simulink model "templatePQreplay"  (R2019b)
settings: Solver=ode23tb  StartTime=0  StopTime=dataSim(l).Time(end)  FixedStep=Ts
model workspace (MAT data in the model file):
  AC8B_test_sdosession : sldodialogs.data.SessionData (value not decoded)
  tp34291882_bceb_4da8_b486_81ba615ab517 = [0 0.0333333 0.0666667 0.1 0.1333334 0.1666667 0.2 0.2333333 0.2666666 0.2999999 0.3333332 0.3666665 ... (13500 elements, 2700x5)]
  tp5fd81924_c6b2_4820_a4c1_c746ac51258e.time = 0
  tp5fd81924_c6b2_4820_a4c1_c746ac51258e.signals(1).values = 0.585108892137
  tp5fd81924_c6b2_4820_a4c1_c746ac51258e.signals(1).dimensions = 1
  tp5fd81924_c6b2_4820_a4c1_c746ac51258e.signals(1).label = 'CSTATE'
  tp5fd81924_c6b2_4820_a4c1_c746ac51258e.signals(1).blockName = 'Unit_I_GAS_AVR_PSS_GOV/General Governor
    | (Continuous)/Break
    | Algebraic
    | Loop /Integrator'
  tp5fd81924_c6b2_4820_a4c1_c746ac51258e.signals(1).stateName = ''
  tp5fd81924_c6b2_4820_a4c1_c746ac51258e.signals(1).inReferencedModel = 0
  tp5fd81924_c6b2_4820_a4c1_c746ac51258e.signals(1).sampleTime = [0 0]
  tp5fd81924_c6b2_4820_a4c1_c746ac51258e.signals(2).values = 0.50266340869
  tp5fd81924_c6b2_4820_a4c1_c746ac51258e.signals(2).dimensions = 1
  tp5fd81924_c6b2_4820_a4c1_c746ac51258e.signals(2).label = 'CSTATE'
  tp5fd81924_c6b2_4820_a4c1_c746ac51258e.signals(2).blockName = 'Unit_I_GAS_AVR_PSS_GOV/General Governor
    | (Continuous)/S0/Integrator'
  tp5fd81924_c6b2_4820_a4c1_c746ac51258e.signals(2).stateName = ''
  tp5fd81924_c6b2_4820_a4c1_c746ac51258e.signals(2).inReferencedModel = 0
  tp5fd81924_c6b2_4820_a4c1_c746ac51258e.signals(2).sampleTime = [0 0]
  tp5fd81924_c6b2_4820_a4c1_c746ac51258e.signals(3).values = -4.9502276038e-07
  tp5fd81924_c6b2_4820_a4c1_c746ac51258e.signals(3).dimensions = 1
  tp5fd81924_c6b2_4820_a4c1_c746ac51258e.signals(3).label = 'CSTATE'
  tp5fd81924_c6b2_4820_a4c1_c746ac51258e.signals(3).blockName = 'Unit_I_GAS_AVR_PSS_GOV/General Governor
    | (Continuous)/S1/S1_TF/Integrator'
  tp5fd81924_c6b2_4820_a4c1_c746ac51258e.signals(3).stateName = ''
  tp5fd81924_c6b2_4820_a4c1_c746ac51258e.signals(3).inReferencedModel = 0
  tp5fd81924_c6b2_4820_a4c1_c746ac51258e.signals(3).sampleTime = [0 0]
  tp5fd81924_c6b2_4820_a4c1_c746ac51258e.signals(4).values = 0.585110202145
  tp5fd81924_c6b2_4820_a4c1_c746ac51258e.signals(4).dimensions = 1
  tp5fd81924_c6b2_4820_a4c1_c746ac51258e.signals(4).label = 'CSTATE'
  tp5fd81924_c6b2_4820_a4c1_c746ac51258e.signals(4).blockName = 'Unit_I_GAS_AVR_PSS_GOV/General Governor
    | (Continuous)/S2/Integrator'
  tp5fd81924_c6b2_4820_a4c1_c746ac51258e.signals(4).stateName = ''
  tp5fd81924_c6b2_4820_a4c1_c746ac51258e.signals(4).inReferencedModel = 0
  tp5fd81924_c6b2_4820_a4c1_c746ac51258e.signals(4).sampleTime = [0 0]
  tp5fd81924_c6b2_4820_a4c1_c746ac51258e.signals(5).values = 0.585108893326
  tp5fd81924_c6b2_4820_a4c1_c746ac51258e.signals(5).dimensions = 1
  tp5fd81924_c6b2_4820_a4c1_c746ac51258e.signals(5).label = 'CSTATE'
  tp5fd81924_c6b2_4820_a4c1_c746ac51258e.signals(5).blockName = 'Unit_I_GAS_AVR_PSS_GOV/General Governor
    | (Continuous)/S3/Integrator'
  tp5fd81924_c6b2_4820_a4c1_c746ac51258e.signals(5).stateName = ''
  tp5fd81924_c6b2_4820_a4c1_c746ac51258e.signals(5).inReferencedModel = 0
  tp5fd81924_c6b2_4820_a4c1_c746ac51258e.signals(5).sampleTime = [0 0]
  tp5fd81924_c6b2_4820_a4c1_c746ac51258e.signals(6).values = 0.502663324956
  tp5fd81924_c6b2_4820_a4c1_c746ac51258e.signals(6).dimensions = 1
  tp5fd81924_c6b2_4820_a4c1_c746ac51258e.signals(6).label = 'CSTATE'
  tp5fd81924_c6b2_4820_a4c1_c746ac51258e.signals(6).blockName = 'Unit_I_GAS_AVR_PSS_GOV/General Governor
    | (Continuous)/S4/Integrator'
  tp5fd81924_c6b2_4820_a4c1_c746ac51258e.signals(6).stateName = ''
  tp5fd81924_c6b2_4820_a4c1_c746ac51258e.signals(6).inReferencedModel = 0
  tp5fd81924_c6b2_4820_a4c1_c746ac51258e.signals(6).sampleTime = [0 0]
  tp5fd81924_c6b2_4820_a4c1_c746ac51258e.signals(7).values = 0.585108883007
  tp5fd81924_c6b2_4820_a4c1_c746ac51258e.signals(7).dimensions = 1
  tp5fd81924_c6b2_4820_a4c1_c746ac51258e.signals(7).label = 'CSTATE'
  tp5fd81924_c6b2_4820_a4c1_c746ac51258e.signals(7).blockName = 'Unit_I_GAS_AVR_PSS_GOV/General Governor
    | (Continuous)/S5/Integrator'
  tp5fd81924_c6b2_4820_a4c1_c746ac51258e.signals(7).stateName = ''
  tp5fd81924_c6b2_4820_a4c1_c746ac51258e.signals(7).inReferencedModel = 0
  tp5fd81924_c6b2_4820_a4c1_c746ac51258e.signals(7).sampleTime = [0 0]
  tp5fd81924_c6b2_4820_a4c1_c746ac51258e.signals(8).values = 0.585108892137
  tp5fd81924_c6b2_4820_a4c1_c746ac51258e.signals(8).dimensions = 1
  tp5fd81924_c6b2_4820_a4c1_c746ac51258e.signals(8).label = 'CSTATE'
  tp5fd81924_c6b2_4820_a4c1_c746ac51258e.signals(8).blockName = 'Unit_I_GAS_AVR_PSS_GOV/General Governor
    | (Continuous)/S6/Integrator'
  tp5fd81924_c6b2_4820_a4c1_c746ac51258e.signals(8).stateName = ''
  tp5fd81924_c6b2_4820_a4c1_c746ac51258e.signals(8).inReferencedModel = 0
  tp5fd81924_c6b2_4820_a4c1_c746ac51258e.signals(8).sampleTime = [0 0]
  tp5fd81924_c6b2_4820_a4c1_c746ac51258e.signals(9).values = 0.0335271378154
  tp5fd81924_c6b2_4820_a4c1_c746ac51258e.signals(9).dimensions = 1
  tp5fd81924_c6b2_4820_a4c1_c746ac51258e.signals(9).label = 'CSTATE'
  tp5fd81924_c6b2_4820_a4c1_c746ac51258e.signals(9).blockName = 'Unit_I_GAS_AVR_PSS_GOV/General Governor
    | (Continuous)/S7/Integrator'
  tp5fd81924_c6b2_4820_a4c1_c746ac51258e.signals(9).stateName = ''
  tp5fd81924_c6b2_4820_a4c1_c746ac51258e.signals(9).inReferencedModel = 0
  tp5fd81924_c6b2_4820_a4c1_c746ac51258e.signals(9).sampleTime = [0 0]
  tp5fd81924_c6b2_4820_a4c1_c746ac51258e.signals(10).values = -1.76344898171e-08
  tp5fd81924_c6b2_4820_a4c1_c746ac51258e.signals(10).dimensions = 1
  tp5fd81924_c6b2_4820_a4c1_c746ac51258e.signals(10).label = 'CSTATE'
  tp5fd81924_c6b2_4820_a4c1_c746ac51258e.signals(10).blockName = 'Unit_I_GAS_AVR_PSS_GOV/General Governor
    | (Continuous)/S8/Integrator'
  tp5fd81924_c6b2_4820_a4c1_c746ac51258e.signals(10).stateName = ''
  tp5fd81924_c6b2_4820_a4c1_c746ac51258e.signals(10).inReferencedModel = 0
  tp5fd81924_c6b2_4820_a4c1_c746ac51258e.signals(10).sampleTime = [0 0]
  tp5fd81924_c6b2_4820_a4c1_c746ac51258e.signals(11).values = 0.585108883007
  tp5fd81924_c6b2_4820_a4c1_c746ac51258e.signals(11).dimensions = 1
  tp5fd81924_c6b2_4820_a4c1_c746ac51258e.signals(11).label = 'CSTATE'
  tp5fd81924_c6b2_4820_a4c1_c746ac51258e.signals(11).blockName = 'Unit_I_GAS_AVR_PSS_GOV/General Governor
    | (Continuous)/S9/Integrator'
  tp5fd81924_c6b2_4820_a4c1_c746ac51258e.signals(11).stateName = ''
  tp5fd81924_c6b2_4820_a4c1_c746ac51258e.signals(11).inReferencedModel = 0
  tp5fd81924_c6b2_4820_a4c1_c746ac51258e.signals(11).sampleTime = [0 0]
  tp5fd81924_c6b2_4820_a4c1_c746ac51258e.signals(12).values = 1.09585681999
  tp5fd81924_c6b2_4820_a4c1_c746ac51258e.signals(12).dimensions = 1
  tp5fd81924_c6b2_4820_a4c1_c746ac51258e.signals(12).label = 'CSTATE'
  tp5fd81924_c6b2_4820_a4c1_c746ac51258e.signals(12).blockName = 'Unit_I_GAS_AVR_PSS_GOV/General Purpose
    | Rotating Excitation System
    | (Continuous)/S0/Tr ~= 0/Integrator'
  tp5fd81924_c6b2_4820_a4c1_c746ac51258e.signals(12).stateName = ''
  tp5fd81924_c6b2_4820_a4c1_c746ac51258e.signals(12).inReferencedModel = 0
  tp5fd81924_c6b2_4820_a4c1_c746ac51258e.signals(12).sampleTime = [0 0]
  tp5fd81924_c6b2_4820_a4c1_c746ac51258e.signals(13).values = -1.11082263543e-06
  tp5fd81924_c6b2_4820_a4c1_c746ac51258e.signals(13).dimensions = 1
  tp5fd81924_c6b2_4820_a4c1_c746ac51258e.signals(13).label = 'CSTATE'
  tp5fd81924_c6b2_4820_a4c1_c746ac51258e.signals(13).blockName = 'Unit_I_GAS_AVR_PSS_GOV/General Purpose
    | Rotating Excitation System
    | (Continuous)/S1/Integrator'
  tp5fd81924_c6b2_4820_a4c1_c746ac51258e.signals(13).stateName = ''
  tp5fd81924_c6b2_4820_a4c1_c746ac51258e.signals(13).inReferencedModel = 0
  tp5fd81924_c6b2_4820_a4c1_c746ac51258e.signals(13).sampleTime = [0 0]
  tp5fd81924_c6b2_4820_a4c1_c746ac51258e.signals(14).values = 0.294440520333
  tp5fd81924_c6b2_4820_a4c1_c746ac51258e.signals(14).dimensions = 1
  tp5fd81924_c6b2_4820_a4c1_c746ac51258e.signals(14).label = 'CSTATE'
  tp5fd81924_c6b2_4820_a4c1_c746ac51258e.signals(14).blockName = 'Unit_I_GAS_AVR_PSS_GOV/General Purpose
    | Rotating Excitation System
    | (Continuous)/S2 + S8/S2/Tb1 ~= 0/Integrator'
  tp5fd81924_c6b2_4820_a4c1_c746ac51258e.signals(14).stateName = ''
  tp5fd81924_c6b2_4820_a4c1_c746ac51258e.signals(14).inReferencedModel = 0
  tp5fd81924_c6b2_4820_a4c1_c746ac51258e.signals(14).sampleTime = [0 0]
  tp5fd81924_c6b2_4820_a4c1_c746ac51258e.signals(15).values = 0.294440505746
  tp5fd81924_c6b2_4820_a4c1_c746ac51258e.signals(15).dimensions = 1
  tp5fd81924_c6b2_4820_a4c1_c746ac51258e.signals(15).label = 'CSTATE'
  tp5fd81924_c6b2_4820_a4c1_c746ac51258e.signals(15).blockName = 'Unit_I_GAS_AVR_PSS_GOV/General Purpose
    | Rotating Excitation System
    | (Continuous)/S2 + S8/S8/Tb2 ~= 0/Integrator'
  tp5fd81924_c6b2_4820_a4c1_c746ac51258e.signals(15).stateName = ''
  tp5fd81924_c6b2_4820_a4c1_c746ac51258e.signals(15).inReferencedModel = 0
  tp5fd81924_c6b2_4820_a4c1_c746ac51258e.signals(15).sampleTime = [0 0]
  tp5fd81924_c6b2_4820_a4c1_c746ac51258e.signals(16).values = 0.29444050528
  tp5fd81924_c6b2_4820_a4c1_c746ac51258e.signals(16).dimensions = 1
  tp5fd81924_c6b2_4820_a4c1_c746ac51258e.signals(16).label = 'CSTATE'
  tp5fd81924_c6b2_4820_a4c1_c746ac51258e.signals(16).blockName = 'Unit_I_GAS_AVR_PSS_GOV/General Purpose
    | Rotating Excitation System
    | (Continuous)/S3/Ta ~= 0/Integrator'
  tp5fd81924_c6b2_4820_a4c1_c746ac51258e.signals(16).stateName = ''
  tp5fd81924_c6b2_4820_a4c1_c746ac51258e.signals(16).inReferencedModel = 0
  tp5fd81924_c6b2_4820_a4c1_c746ac51258e.signals(16).sampleTime = [0 0]
  tp5fd81924_c6b2_4820_a4c1_c746ac51258e.signals(17).values = 1.17292432998
  tp5fd81924_c6b2_4820_a4c1_c746ac51258e.signals(17).dimensions = 1
  tp5fd81924_c6b2_4820_a4c1_c746ac51258e.signals(17).label = 'CSTATE'
  tp5fd81924_c6b2_4820_a4c1_c746ac51258e.signals(17).blockName = 'Unit_I_GAS_AVR_PSS_GOV/General Purpose
    | Rotating Excitation System
    | (Continuous)/S4/Tf2 ~= 0/Integrator'
  tp5fd81924_c6b2_4820_a4c1_c746ac51258e.signals(17).stateName = ''
  tp5fd81924_c6b2_4820_a4c1_c746ac51258e.signals(17).inReferencedModel = 0
  tp5fd81924_c6b2_4820_a4c1_c746ac51258e.signals(17).sampleTime = [0 0]
  tp5fd81924_c6b2_4820_a4c1_c746ac51258e.signals(18).values = 1.17292433904
  tp5fd81924_c6b2_4820_a4c1_c746ac51258e.signals(18).dimensions = 1
  tp5fd81924_c6b2_4820_a4c1_c746ac51258e.signals(18).label = 'CSTATE'
  tp5fd81924_c6b2_4820_a4c1_c746ac51258e.signals(18).blockName = 'Unit_I_GAS_AVR_PSS_GOV/General Purpose
    | Rotating Excitation System
    | (Continuous)/S5/Integrator'
  tp5fd81924_c6b2_4820_a4c1_c746ac51258e.signals(18).stateName = ''
  tp5fd81924_c6b2_4820_a4c1_c746ac51258e.signals(18).inReferencedModel = 0
  tp5fd81924_c6b2_4820_a4c1_c746ac51258e.signals(18).sampleTime = [0 0]
  tp5fd81924_c6b2_4820_a4c1_c746ac51258e.signals(19).values = -0.299278194471
  tp5fd81924_c6b2_4820_a4c1_c746ac51258e.signals(19).dimensions = 1
  tp5fd81924_c6b2_4820_a4c1_c746ac51258e.signals(19).label = 'CSTATE'
  tp5fd81924_c6b2_4820_a4c1_c746ac51258e.signals(19).blockName = 'Unit_I_GAS_AVR_PSS_GOV/General Purpose
    | Rotating Excitation System
    | (Continuous)/S6/Integrator'
  tp5fd81924_c6b2_4820_a4c1_c746ac51258e.signals(19).stateName = ''
  tp5fd81924_c6b2_4820_a4c1_c746ac51258e.signals(19).inReferencedModel = 0
  tp5fd81924_c6b2_4820_a4c1_c746ac51258e.signals(19).sampleTime = [0 0]
  tp5fd81924_c6b2_4820_a4c1_c746ac51258e.signals(20).values = 1.50129144782
  tp5fd81924_c6b2_4820_a4c1_c746ac51258e.signals(20).dimensions = 1
  tp5fd81924_c6b2_4820_a4c1_c746ac51258e.signals(20).label = 'CSTATE'
  tp5fd81924_c6b2_4820_a4c1_c746ac51258e.signals(20).blockName = 'Unit_I_GAS_AVR_PSS_GOV/General Purpose
    | Rotating Excitation System
    | (Continuous)/S7/Integrator'
  tp5fd81924_c6b2_4820_a4c1_c746ac51258e.signals(20).stateName = ''
  tp5fd81924_c6b2_4820_a4c1_c746ac51258e.signals(20).inReferencedModel = 0
  tp5fd81924_c6b2_4820_a4c1_c746ac51258e.signals(20).sampleTime = [0 0]
  tp5fd81924_c6b2_4820_a4c1_c746ac51258e.signals(21).values = 1.17292433193
  tp5fd81924_c6b2_4820_a4c1_c746ac51258e.signals(21).dimensions = 1
  tp5fd81924_c6b2_4820_a4c1_c746ac51258e.signals(21).label = 'CSTATE'
  tp5fd81924_c6b2_4820_a4c1_c746ac51258e.signals(21).blockName = 'Unit_I_GAS_AVR_PSS_GOV/General Purpose
    | Rotating Excitation System
    | (Continuous)/S9/Tp ~= 0/Integrator'
  tp5fd81924_c6b2_4820_a4c1_c746ac51258e.signals(21).stateName = ''
  tp5fd81924_c6b2_4820_a4c1_c746ac51258e.signals(21).inReferencedModel = 0
  tp5fd81924_c6b2_4820_a4c1_c746ac51258e.signals(21).sampleTime = [0 0]
  tp5fd81924_c6b2_4820_a4c1_c746ac51258e.signals(22).values = -1.49881455181e-10
  tp5fd81924_c6b2_4820_a4c1_c746ac51258e.signals(22).dimensions = 1
  tp5fd81924_c6b2_4820_a4c1_c746ac51258e.signals(22).label = 'CSTATE'
  tp5fd81924_c6b2_4820_a4c1_c746ac51258e.signals(22).blockName = 'Unit_I_GAS_AVR_PSS_GOV/Power System
    | Stabilizer 2A
    | (Continuous)/Ramp-Tracking Filter/T9 ~= 0/Filter1/TF1/Integrator'
  tp5fd81924_c6b2_4820_a4c1_c746ac51258e.signals(22).stateName = ''
  tp5fd81924_c6b2_4820_a4c1_c746ac51258e.signals(22).inReferencedModel = 0
  tp5fd81924_c6b2_4820_a4c1_c746ac51258e.signals(22).sampleTime = [0 0]
  tp5fd81924_c6b2_4820_a4c1_c746ac51258e.signals(23).values = -1.50085906522e-10
  tp5fd81924_c6b2_4820_a4c1_c746ac51258e.signals(23).dimensions = 1
  tp5fd81924_c6b2_4820_a4c1_c746ac51258e.signals(23).label = 'CSTATE'
  tp5fd81924_c6b2_4820_a4c1_c746ac51258e.signals(23).blockName = 'Unit_I_GAS_AVR_PSS_GOV/Power System
    | Stabilizer 2A
    | (Continuous)/Ramp-Tracking Filter/T9 ~= 0/Filter1/TF2/Integrator'
  tp5fd81924_c6b2_4820_a4c1_c746ac51258e.signals(23).stateName = ''
  tp5fd81924_c6b2_4820_a4c1_c746ac51258e.signals(23).inReferencedModel = 0
  tp5fd81924_c6b2_4820_a4c1_c746ac51258e.signals(23).sampleTime = [0 0]
  tp5fd81924_c6b2_4820_a4c1_c746ac51258e.signals(24).values = -1.50034793802e-10
  tp5fd81924_c6b2_4820_a4c1_c746ac51258e.signals(24).dimensions = 1
  tp5fd81924_c6b2_4820_a4c1_c746ac51258e.signals(24).label = 'CSTATE'
  tp5fd81924_c6b2_4820_a4c1_c746ac51258e.signals(24).blockName = 'Unit_I_GAS_AVR_PSS_GOV/Power System
    | Stabilizer 2A
    | (Continuous)/Ramp-Tracking Filter/T9 ~= 0/Filter1/TF3/Integrator'
  tp5fd81924_c6b2_4820_a4c1_c746ac51258e.signals(24).stateName = ''
  tp5fd81924_c6b2_4820_a4c1_c746ac51258e.signals(24).inReferencedModel = 0
  tp5fd81924_c6b2_4820_a4c1_c746ac51258e.signals(24).sampleTime = [0 0]
  tp5fd81924_c6b2_4820_a4c1_c746ac51258e.signals(25).values = -1.49983681133e-10
  tp5fd81924_c6b2_4820_a4c1_c746ac51258e.signals(25).dimensions = 1
  tp5fd81924_c6b2_4820_a4c1_c746ac51258e.signals(25).label = 'CSTATE'
  tp5fd81924_c6b2_4820_a4c1_c746ac51258e.signals(25).blockName = 'Unit_I_GAS_AVR_PSS_GOV/Power System
    | Stabilizer 2A
    | (Continuous)/Ramp-Tracking Filter/T9 ~= 0/Filter1/TF4/Integrator'
  tp5fd81924_c6b2_4820_a4c1_c746ac51258e.signals(25).stateName = ''
  tp5fd81924_c6b2_4820_a4c1_c746ac51258e.signals(25).inReferencedModel = 0
  tp5fd81924_c6b2_4820_a4c1_c746ac51258e.signals(25).sampleTime = [0 0]
  tp5fd81924_c6b2_4820_a4c1_c746ac51258e.signals(26).values = -1.49932568515e-10
  tp5fd81924_c6b2_4820_a4c1_c746ac51258e.signals(26).dimensions = 1
  tp5fd81924_c6b2_4820_a4c1_c746ac51258e.signals(26).label = 'CSTATE'
  tp5fd81924_c6b2_4820_a4c1_c746ac51258e.signals(26).blockName = 'Unit_I_GAS_AVR_PSS_GOV/Power System
    | Stabilizer 2A
    | (Continuous)/Ramp-Tracking Filter/T9 ~= 0/Filter1/TF5/Integrator'
  tp5fd81924_c6b2_4820_a4c1_c746ac51258e.signals(26).stateName = ''
  tp5fd81924_c6b2_4820_a4c1_c746ac51258e.signals(26).inReferencedModel = 0
  tp5fd81924_c6b2_4820_a4c1_c746ac51258e.signals(26).sampleTime = [0 0]
  tp5fd81924_c6b2_4820_a4c1_c746ac51258e.signals(27).values = -1.76344805856e-08
  tp5fd81924_c6b2_4820_a4c1_c746ac51258e.signals(27).dimensions = 1
  tp5fd81924_c6b2_4820_a4c1_c746ac51258e.signals(27).label = 'CSTATE'
  tp5fd81924_c6b2_4820_a4c1_c746ac51258e.signals(27).blockName = 'Unit_I_GAS_AVR_PSS_GOV/Power System
    | Stabilizer 2A
    | (Continuous)/S0/Integrator'
  tp5fd81924_c6b2_4820_a4c1_c746ac51258e.signals(27).stateName = ''
  tp5fd81924_c6b2_4820_a4c1_c746ac51258e.signals(27).inReferencedModel = 0
  tp5fd81924_c6b2_4820_a4c1_c746ac51258e.signals(27).sampleTime = [0 0]
  tp5fd81924_c6b2_4820_a4c1_c746ac51258e.signals(28).values = 1.49872449229e-10
  tp5fd81924_c6b2_4820_a4c1_c746ac51258e.signals(28).dimensions = 1
  tp5fd81924_c6b2_4820_a4c1_c746ac51258e.signals(28).label = 'CSTATE'
  tp5fd81924_c6b2_4820_a4c1_c746ac51258e.signals(28).blockName = 'Unit_I_GAS_AVR_PSS_GOV/Power System
    | Stabilizer 2A
    | (Continuous)/S1/Tw2 ~= 0/Integrator'
  tp5fd81924_c6b2_4820_a4c1_c746ac51258e.signals(28).stateName = ''
  tp5fd81924_c6b2_4820_a4c1_c746ac51258e.signals(28).inReferencedModel = 0
  tp5fd81924_c6b2_4820_a4c1_c746ac51258e.signals(28).sampleTime = [0 0]
  tp5fd81924_c6b2_4820_a4c1_c746ac51258e.signals(29).values = -4.09162771813e-09
  tp5fd81924_c6b2_4820_a4c1_c746ac51258e.signals(29).dimensions = 1
  tp5fd81924_c6b2_4820_a4c1_c746ac51258e.signals(29).label = 'CSTATE'
  tp5fd81924_c6b2_4820_a4c1_c746ac51258e.signals(29).blockName = 'Unit_I_GAS_AVR_PSS_GOV/Power System
    | Stabilizer 2A
    | (Continuous)/S18/Tb ~= 0/Integrator'
  tp5fd81924_c6b2_4820_a4c1_c746ac51258e.signals(29).stateName = ''
  tp5fd81924_c6b2_4820_a4c1_c746ac51258e.signals(29).inReferencedModel = 0
  tp5fd81924_c6b2_4820_a4c1_c746ac51258e.signals(29).sampleTime = [0 0]
  tp5fd81924_c6b2_4820_a4c1_c746ac51258e.signals(30).values = -1.49882113433e-10
  tp5fd81924_c6b2_4820_a4c1_c746ac51258e.signals(30).dimensions = 1
  tp5fd81924_c6b2_4820_a4c1_c746ac51258e.signals(30).label = 'CSTATE'
  tp5fd81924_c6b2_4820_a4c1_c746ac51258e.signals(30).blockName = 'Unit_I_GAS_AVR_PSS_GOV/Power System
    | Stabilizer 2A
    | (Continuous)/S2/T6 ~= 0/Integrator'
  tp5fd81924_c6b2_4820_a4c1_c746ac51258e.signals(30).stateName = ''
  tp5fd81924_c6b2_4820_a4c1_c746ac51258e.signals(30).inReferencedModel = 0
  tp5fd81924_c6b2_4820_a4c1_c746ac51258e.signals(30).sampleTime = [0 0]
  tp5fd81924_c6b2_4820_a4c1_c746ac51258e.signals(31).values = 0.502663409208
  tp5fd81924_c6b2_4820_a4c1_c746ac51258e.signals(31).dimensions = 1
  tp5fd81924_c6b2_4820_a4c1_c746ac51258e.signals(31).label = 'CSTATE'
  tp5fd81924_c6b2_4820_a4c1_c746ac51258e.signals(31).blockName = 'Unit_I_GAS_AVR_PSS_GOV/Power System
    | Stabilizer 2A
    | (Continuous)/S3/Integrator'
  tp5fd81924_c6b2_4820_a4c1_c746ac51258e.signals(31).stateName = ''
  tp5fd81924_c6b2_4820_a4c1_c746ac51258e.signals(31).inReferencedModel = 0
  tp5fd81924_c6b2_4820_a4c1_c746ac51258e.signals(31).sampleTime = [0 0]
  tp5fd81924_c6b2_4820_a4c1_c746ac51258e.signals(32).values = -6.11813281183e-12
  tp5fd81924_c6b2_4820_a4c1_c746ac51258e.signals(32).dimensions = 1
  tp5fd81924_c6b2_4820_a4c1_c746ac51258e.signals(32).label = 'CSTATE'
  tp5fd81924_c6b2_4820_a4c1_c746ac51258e.signals(32).blockName = 'Unit_I_GAS_AVR_PSS_GOV/Power System
    | Stabilizer 2A
    | (Continuous)/S4/Tw4 ~= 0/Integrator'
  tp5fd81924_c6b2_4820_a4c1_c746ac51258e.signals(32).stateName = ''
  tp5fd81924_c6b2_4820_a4c1_c746ac51258e.signals(32).inReferencedModel = 0
  tp5fd81924_c6b2_4820_a4c1_c746ac51258e.signals(32).sampleTime = [0 0]
  tp5fd81924_c6b2_4820_a4c1_c746ac51258e.signals(33).values = 6.57485586185e-16
  tp5fd81924_c6b2_4820_a4c1_c746ac51258e.signals(33).dimensions = 1
  tp5fd81924_c6b2_4820_a4c1_c746ac51258e.signals(33).label = 'CSTATE'
  tp5fd81924_c6b2_4820_a4c1_c746ac51258e.signals(33).blockName = 'Unit_I_GAS_AVR_PSS_GOV/Power System
    | Stabilizer 2A
    | (Continuous)/S5/T7 ~= 0/Integrator'
  tp5fd81924_c6b2_4820_a4c1_c746ac51258e.signals(33).stateName = ''
  tp5fd81924_c6b2_4820_a4c1_c746ac51258e.signals(33).inReferencedModel = 0
  tp5fd81924_c6b2_4820_a4c1_c746ac51258e.signals(33).sampleTime = [0 0]
  tp5fd81924_c6b2_4820_a4c1_c746ac51258e.signals(34).values = -4.09146911874e-09
  tp5fd81924_c6b2_4820_a4c1_c746ac51258e.signals(34).dimensions = 1
  tp5fd81924_c6b2_4820_a4c1_c746ac51258e.signals(34).label = 'CSTATE'
  tp5fd81924_c6b2_4820_a4c1_c746ac51258e.signals(34).blockName = 'Unit_I_GAS_AVR_PSS_GOV/Power System
    | Stabilizer 2A
    | (Continuous)/S6/T2 ~= 0/Integrator'
  tp5fd81924_c6b2_4820_a4c1_c746ac51258e.signals(34).stateName = ''
  tp5fd81924_c6b2_4820_a4c1_c746ac51258e.signals(34).inReferencedModel = 0
  tp5fd81924_c6b2_4820_a4c1_c746ac51258e.signals(34).sampleTime = [0 0]
  tp5fd81924_c6b2_4820_a4c1_c746ac51258e.signals(35).values = -4.09167395604e-09
  tp5fd81924_c6b2_4820_a4c1_c746ac51258e.signals(35).dimensions = 1
  tp5fd81924_c6b2_4820_a4c1_c746ac51258e.signals(35).label = 'CSTATE'
  tp5fd81924_c6b2_4820_a4c1_c746ac51258e.signals(35).blockName = 'Unit_I_GAS_AVR_PSS_GOV/Power System
    | Stabilizer 2A
    | (Continuous)/S7/T4 ~= 0/Integrator'
  tp5fd81924_c6b2_4820_a4c1_c746ac51258e.signals(35).stateName = ''
  tp5fd81924_c6b2_4820_a4c1_c746ac51258e.signals(35).inReferencedModel = 0
  tp5fd81924_c6b2_4820_a4c1_c746ac51258e.signals(35).sampleTime = [0 0]
  tp5fd81924_c6b2_4820_a4c1_c746ac51258e.signals(36).values = 0.001094934692
  tp5fd81924_c6b2_4820_a4c1_c746ac51258e.signals(36).dimensions = 1
  tp5fd81924_c6b2_4820_a4c1_c746ac51258e.signals(36).label = 'CSTATE'
  tp5fd81924_c6b2_4820_a4c1_c746ac51258e.signals(36).blockName = 'Unit_I_GAS_AVR_PSS_GOV/Subsystem/Three-Phase
    | Dynamic Load/Model/ filter1'
  tp5fd81924_c6b2_4820_a4c1_c746ac51258e.signals(36).stateName = ''
  tp5fd81924_c6b2_4820_a4c1_c746ac51258e.signals(36).inReferencedModel = 0
  tp5fd81924_c6b2_4820_a4c1_c746ac51258e.signals(36).sampleTime = [0 0]
  tp5fd81924_c6b2_4820_a4c1_c746ac51258e.signals(37).values = 0.187748964781
  tp5fd81924_c6b2_4820_a4c1_c746ac51258e.signals(37).dimensions = 1
  tp5fd81924_c6b2_4820_a4c1_c746ac51258e.signals(37).label = 'CSTATE'
  tp5fd81924_c6b2_4820_a4c1_c746ac51258e.signals(37).blockName = 'Unit_I_GAS_AVR_PSS_GOV/Subsystem/Three-Phase
    | Dynamic Load/Model/Break 
    | Alg. Loop I1/imag/State Space'
  tp5fd81924_c6b2_4820_a4c1_c746ac51258e.signals(37).stateName = ''
  tp5fd81924_c6b2_4820_a4c1_c746ac51258e.signals(37).inReferencedModel = 0
  tp5fd81924_c6b2_4820_a4c1_c746ac51258e.signals(37).sampleTime = [0 0]
  tp5fd81924_c6b2_4820_a4c1_c746ac51258e.signals(38).values = -0.851179474107
  tp5fd81924_c6b2_4820_a4c1_c746ac51258e.signals(38).dimensions = 1
  tp5fd81924_c6b2_4820_a4c1_c746ac51258e.signals(38).label = 'CSTATE'
  tp5fd81924_c6b2_4820_a4c1_c746ac51258e.signals(38).blockName = 'Unit_I_GAS_AVR_PSS_GOV/Subsystem/Three-Phase
    | Dynamic Load/Model/Break 
    | Alg. Loop I1/real/State Space'
  tp5fd81924_c6b2_4820_a4c1_c746ac51258e.signals(38).stateName = ''
  tp5fd81924_c6b2_4820_a4c1_c746ac51258e.signals(38).inReferencedModel = 0
  tp5fd81924_c6b2_4820_a4c1_c746ac51258e.signals(38).sampleTime = [0 0]
  tp5fd81924_c6b2_4820_a4c1_c746ac51258e.signals(39).values = 0
  tp5fd81924_c6b2_4820_a4c1_c746ac51258e.signals(39).dimensions = 1
  tp5fd81924_c6b2_4820_a4c1_c746ac51258e.signals(39).label = 'CSTATE'
  tp5fd81924_c6b2_4820_a4c1_c746ac51258e.signals(39).blockName = 'Unit_I_GAS_AVR_PSS_GOV/Synchronous Machine
    | pu Standard/Electrical model/Integrator'
  tp5fd81924_c6b2_4820_a4c1_c746ac51258e.signals(39).stateName = ''
  tp5fd81924_c6b2_4820_a4c1_c746ac51258e.signals(39).inReferencedModel = 0
  tp5fd81924_c6b2_4820_a4c1_c746ac51258e.signals(39).sampleTime = [0 0]
  tp5fd81924_c6b2_4820_a4c1_c746ac51258e.signals(40).values = 1.54599756848
  tp5fd81924_c6b2_4820_a4c1_c746ac51258e.signals(40).dimensions = 1
  tp5fd81924_c6b2_4820_a4c1_c746ac51258e.signals(40).label = 'CSTATE'
  tp5fd81924_c6b2_4820_a4c1_c746ac51258e.signals(40).blockName = 'Unit_I_GAS_AVR_PSS_GOV/Synchronous Machine
    | pu Standard/Electrical model/Synchronous Machine
    | Continuous Model/Saturation/Lmd_sat/Time Constant/Integrator'
  tp5fd81924_c6b2_4820_a4c1_c746ac51258e.signals(40).stateName = ''
  tp5fd81924_c6b2_4820_a4c1_c746ac51258e.signals(40).inReferencedModel = 0
  tp5fd81924_c6b2_4820_a4c1_c746ac51258e.signals(40).sampleTime = [0 0]
  tp5fd81924_c6b2_4820_a4c1_c746ac51258e.signals(41).values = 1.17520536613
  tp5fd81924_c6b2_4820_a4c1_c746ac51258e.signals(41).dimensions = 1
  tp5fd81924_c6b2_4820_a4c1_c746ac51258e.signals(41).label = 'CSTATE'
  tp5fd81924_c6b2_4820_a4c1_c746ac51258e.signals(41).blockName = 'Unit_I_GAS_AVR_PSS_GOV/Synchronous Machine
    | pu Standard/Electrical model/Synchronous Machine
    | Continuous Model/Saturation/Lmq_sat/Time Constant/Integrator'
  tp5fd81924_c6b2_4820_a4c1_c746ac51258e.signals(41).stateName = ''
  tp5fd81924_c6b2_4820_a4c1_c746ac51258e.signals(41).inReferencedModel = 0
  tp5fd81924_c6b2_4820_a4c1_c746ac51258e.signals(41).sampleTime = [0 0]
  tp5fd81924_c6b2_4820_a4c1_c746ac51258e.signals(42).values = [-0.518031918821 0.967243110439 1.36455540141 0.99548410429 -0.468302992918 -0.468302992663]
  tp5fd81924_c6b2_4820_a4c1_c746ac51258e.signals(42).dimensions = 6
  tp5fd81924_c6b2_4820_a4c1_c746ac51258e.signals(42).label = 'CSTATE'
  tp5fd81924_c6b2_4820_a4c1_c746ac51258e.signals(42).blockName = 'Unit_I_GAS_AVR_PSS_GOV/Synchronous Machine
    | pu Standard/Electrical model/Synchronous Machine
    | Continuous Model/phi/Integrator'
  tp5fd81924_c6b2_4820_a4c1_c746ac51258e.signals(42).stateName = ''
  tp5fd81924_c6b2_4820_a4c1_c746ac51258e.signals(42).inReferencedModel = 0
  tp5fd81924_c6b2_4820_a4c1_c746ac51258e.signals(42).sampleTime = [0 0]
  tp5fd81924_c6b2_4820_a4c1_c746ac51258e.signals(43).values = [-4.97692287468e-11 -1.28297588951e-11]
  tp5fd81924_c6b2_4820_a4c1_c746ac51258e.signals(43).dimensions = 2
  tp5fd81924_c6b2_4820_a4c1_c746ac51258e.signals(43).label = 'CSTATE'
  tp5fd81924_c6b2_4820_a4c1_c746ac51258e.signals(43).blockName = 'Unit_I_GAS_AVR_PSS_GOV/Synchronous Machine
    | pu Standard/Electrical model/Vd1 Vq1, I2/Vdq2->Idq2/Integrator'
  tp5fd81924_c6b2_4820_a4c1_c746ac51258e.signals(43).stateName = ''
  tp5fd81924_c6b2_4820_a4c1_c746ac51258e.signals(43).inReferencedModel = 0
  tp5fd81924_c6b2_4820_a4c1_c746ac51258e.signals(43).sampleTime = [0 0]
  tp5fd81924_c6b2_4820_a4c1_c746ac51258e.signals(44).values = -1.76344902498e-08
  tp5fd81924_c6b2_4820_a4c1_c746ac51258e.signals(44).dimensions = 1
  tp5fd81924_c6b2_4820_a4c1_c746ac51258e.signals(44).label = 'CSTATE'
  tp5fd81924_c6b2_4820_a4c1_c746ac51258e.signals(44).blockName = 'Unit_I_GAS_AVR_PSS_GOV/Synchronous Machine
    | pu Standard/Mechanical model/Integrator'
  tp5fd81924_c6b2_4820_a4c1_c746ac51258e.signals(44).stateName = ''
  tp5fd81924_c6b2_4820_a4c1_c746ac51258e.signals(44).inReferencedModel = 0
  tp5fd81924_c6b2_4820_a4c1_c746ac51258e.signals(44).sampleTime = [0 0]
  tp5fd81924_c6b2_4820_a4c1_c746ac51258e.signals(45).values = -1.57079632679
  tp5fd81924_c6b2_4820_a4c1_c746ac51258e.signals(45).dimensions = 1
  tp5fd81924_c6b2_4820_a4c1_c746ac51258e.signals(45).label = 'CSTATE'
  tp5fd81924_c6b2_4820_a4c1_c746ac51258e.signals(45).blockName = 'Unit_I_GAS_AVR_PSS_GOV/Synchronous Machine
    | pu Standard/Mechanical model/Integrator1'
  tp5fd81924_c6b2_4820_a4c1_c746ac51258e.signals(45).stateName = ''
  tp5fd81924_c6b2_4820_a4c1_c746ac51258e.signals(45).inReferencedModel = 0
  tp5fd81924_c6b2_4820_a4c1_c746ac51258e.signals(45).sampleTime = [0 0]
  tp5fd81924_c6b2_4820_a4c1_c746ac51258e.signals(46).values = -1.25934669875
  tp5fd81924_c6b2_4820_a4c1_c746ac51258e.signals(46).dimensions = 1
  tp5fd81924_c6b2_4820_a4c1_c746ac51258e.signals(46).label = 'CSTATE'
  tp5fd81924_c6b2_4820_a4c1_c746ac51258e.signals(46).blockName = 'Unit_I_GAS_AVR_PSS_GOV/Synchronous Machine
    | pu Standard/Mechanical model/Integrator2'
  tp5fd81924_c6b2_4820_a4c1_c746ac51258e.signals(46).stateName = ''
  tp5fd81924_c6b2_4820_a4c1_c746ac51258e.signals(46).inReferencedModel = 0
  tp5fd81924_c6b2_4820_a4c1_c746ac51258e.signals(46).sampleTime = [0 0]
  tp61e2f470_2812_498a_af75_e87b8b944307 = [0 0.0333333 0.0666667 0.1 0.1333334 0.1666667 0.2 0.2333333 0.2666666 0.2999999 0.3333332 0.3666665 ... (13500 elements, 2700x5)]
  tpfa3056f0_c430_45b3_969f_b76cef1498ad : object (value not decoded)
undefined symbols (not defined in the file): dataSim, dyn, Fnom, g, gcbh, genTpd0, genTppd0, genTppq0, genTpq0, genXd, genXl, genXpd, genXppd, genXppq, genXpq, genXq, govDisable, ifd, init, j, l, p, Psnubber, Rsnubber, sps_rtmsupport, sys, Tb1, Tc1, Vnom, vt
libraries: powerlib x32, modelLibrary x22, simulink x15, powerlib_meascontrol x6, spsST2AModel x4, GenLib x2
(part 1 of 4)
settings Model: SimulationMode=accelerator  TunableVars=avrE1,avrE2,avrFbf,avrFlimf,avrKc,avrKd,avrKe,avrKefd,avrKf,avrKh,avrKii,avrKip,avrKvi,avrKvp,avrKvphz,avrLimflg,avrNvphz,avrRcomp,avrSe1,avrSe2,avrTa,avrTb1,avrTb2,avrTc1,avrTc2,avrTe,avrTf,avrTf1,avrTf2,avrTp,avrTr,avrVcmax,avrVfmax,avrVfmin,avrVimax,avrVrmax,avrVrmin,avrXc,avrXcomp,genD,genH,genKis,genPfd,genPfq,genPkd,genPkq,genRa,genRcomp,genS1,genS12,genSpeed,genTpd0,genTppd0,genTppq0,genTpq0,genXcomp,genXd,genXl,genXpd,genXppd,genXppq,genXpq,genXq,govAsest,govAset,govDb,govDm,govFlag,govKa,govKdgov,govKigov,govKiload,govKimw,govKpgov,govKpload,govKturb,govLdref,govMaxerr,govMinerr,govPmwset,govR,govRclose,govRdown,govRopen,govRselect,govRup,govTa,govTact,govTb,govTc,govTdgov,govTeng,govTfload,govTpelec,govTsa,govTsb,govVmax,govVmin,govWfnl,pssA,pssJ1,pssJ2,pssK1,pssK2,pssKs1,pssKs2,pssKs3,pssKs4,pssM,pssN,pssT1,pssT2,pssT3,pssT4,pssT6,pssT7,pssT8,pssT9,pssTa,pssTb,pssTw1,pssTw2,pssTw3,pssTw4,pssVstmax,pssVstmin  TunableVarsStorageClass=Auto,Auto,Auto,Auto,Auto,Auto,Auto,Auto,Auto,Auto,Auto,Auto,Auto,Auto,Auto,Auto,Auto,Auto,Auto,Auto,Auto,Auto,Auto,Auto,Auto,Auto,Auto,Auto,Auto,Auto,Auto,Auto,Auto,Auto,Auto,Auto,Auto,Auto,Auto,Auto,Auto,Auto,Auto,Auto,Auto,Auto,Auto,Auto,Auto,Auto,Auto,Auto,Auto,Auto,Auto,Auto,Auto,Auto,Auto,Auto,Auto,Auto,Auto,Auto,Auto,Auto,Auto,Auto,Auto,Auto,Auto,Auto,Auto,Auto,Auto,Auto,Auto,Auto,Auto,Auto,Auto,Auto,Auto,Auto,Auto,Auto,Auto,Auto,Auto,Auto,Auto,Auto,Auto,Auto,Auto,Auto,Auto,Auto,Auto,Auto,Auto,Auto,Auto,Auto,Auto,Auto,Auto,Auto,Auto,Auto,Auto,Auto,Auto,Auto,Auto,Auto,Auto,Auto,Auto,Auto,Auto,Auto,Auto,Auto,Auto,Auto  TunableVarsTypeQualifier=,,,,,,,,,,,,,,,,,,,,,,,,,,,,,,,,,,,,,,,,,,,,,,,,,,,,,,,,,,,,,,,,,,,,,,,,,,,,,,,,,,,,,,,,,,,,,,,,,,,,,,,,,,,,,,,,,,,,,,,,,,,,,  Creator=cosorio  LastModifiedBy=gdudgeon
settings SolverCC: AutoInsertRateTranBlk=on
settings DataIOCC: ExternalInput=Exp(l).InputData  InitialState=getstatestruct(op(l))  LoadExternalInput=on  LoadInitialState=on  SaveFormat=StructureWithTime  SignalLogging=off  DSMLogging=off  SaveTime=off  ReturnWorkspaceOutputs=off  ReturnWorkspaceOutputsName=SDOSimTest_Log
settings OptimizationCC: BlockReduction=off  BooleanDataType=off  BufferReuse=off  LifeSpan=inf
settings DebuggingCC: AlgebraicLoopMsg=none  SaveWithParameterizedLinksMsg=none  UnderspecifiedInitializationDetection=Classic  MergeDetectMultiDrivingBlocksExec=none  SignalResolutionControl=None  IgnoredZcDiagnostic=none  UnconnectedInputMsg=none  UnconnectedOutputMsg=none  UnconnectedLineMsg=none  AllowSymbolicDim=off  ModelReferenceExtraNoncontSigs=none  SFUnexpectedBacktrackingDiag=warning  SFNoUnconditionalDefaultTransitionDiag=warning  SFExecutionAtInitializationDiag=none  ArithmeticOperatorsInVariantConditions=warning
settings HardwareCC: ProdBitPerPointer=32  ProdBitPerSizeT=32  ProdBitPerPtrDiffT=32  ProdLargestAtomicFloat=None  ProdIntDivRoundTo=Undefined  ProdEndianess=Unspecified  ProdWordSize=32  ProdHWDeviceType=32-bit Generic  TargetUnknown=on
settings ModelReferenceCC: PropagateSignalLabelsOutOfModel=off
settings SFSimCC: SimUseLocalCustomCode=off  CustomCodeUndefinedFunction=UseInterfaceOnly
settings RTWCC: RTWUseLocalCustomCode=off
settings CodeAppCC: StateflowObjectComments=on
settings GRTTargetCC: TargetLangStandard=C89/C90 (ANSI)  GeneratePreprocessorConditionals=Disable all
settings ConfigComp: CovMetricSettings=dw  CovHtmlReporting=on  CovSaveCumulativeToWorkspaceVar=on  CovSaveSingleToWorkspaceVar=on  CovExternalEMLEnable=off  CovSFcnEnable=off
settings SimscapeCC: SimscapeNormalizeSystem=off

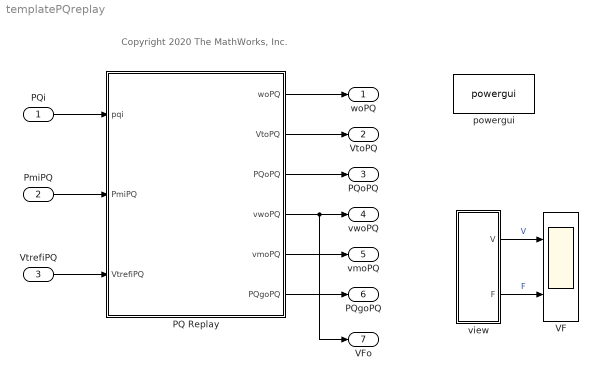
== system templatePQreplay ==
  note: Copyright 2020 The MathWorks, Inc.
  PQi : Inport
  PmiPQ : Inport  Port=2
  VtrefiPQ : Inport  Port=3
  PQ Replay : Subsystem
      mask Display: disp('{\bf\fontsize{20} PQ Replay}', 'texmode','on');
  VF : Scope  NumInputPorts=2
  powergui : powerlib/powergui  Priority=1  SimulationMode=Phasor  SampleTime=50e-6  frequency=60  Iterations=50  frequencyindice=60  Pbase=100e6  ErrMax=1e-4  UnitsV=kV  UnitsW=MW  buscounter=0  FunctionMessages=off  echomessages=off  EnableUseOfTLC=off  CurrentSourceSwitches=off  DisableSnubberDevices=off  DisableRonSwitches=off  DisableVfSwitches=off  DisplayEquations=off  AutomaticDiscreteSolvers=off  SolverType=Tustin/Backward Euler (TBE)  Interpol=off  ExternalGateDelay=off  methode=off  Ts=100  x0status=blocks  SPID=on  SwTol=0  HookPort=off  NonlinearTolerance=0  nMaxIteration=15  ContinueOnMaxIteration=off  RestoreLinks=warning  ResistiveCurrentMeasurement=off  Frange=[0:2:500]  Ylog=off  Xlog=on  ShowGrid=off  save=off  variable=ZData  structure=0  ZoomFFT=off  StartTime=0.0  cycles=1  DisplayStyle=1  fundamental=60  FreqAxis=off  MaxFrequency=1000  frequencyindicesteady=1  RmsSteady=1  display=off
      settings: SourceProductName=Simscape Electrical
  view : Subsystem
  woPQ : Outport  VectorParamsAs1DForOutWhenUnconnected=off
  VtoPQ : Outport  Port=2  VectorParamsAs1DForOutWhenUnconnected=off
  PQoPQ : Outport  Port=3  SampleTime=1/30  VectorParamsAs1DForOutWhenUnconnected=off
  vwoPQ : Outport  Port=4  VectorParamsAs1DForOutWhenUnconnected=off
  vmoPQ : Outport  Port=5  VectorParamsAs1DForOutWhenUnconnected=off
  PQgoPQ : Outport  Port=6  SampleTime=1/30  VectorParamsAs1DForOutWhenUnconnected=off
  VFo : Outport  Port=7  SampleTime=1/30  VectorParamsAs1DForOutWhenUnconnected=off
  wires:
  PQi/1 -> PQ Replay/1(pqi)
  PQ Replay/1(woPQ) -> woPQ/1
  PQ Replay/2(VtoPQ) -> VtoPQ/1
  PQ Replay/3(PQoPQ) -> PQoPQ/1
  PQ Replay/4(vwoPQ) -> VFo/1, vwoPQ/1
  PQ Replay/5(vmoPQ) -> vmoPQ/1
  PQ Replay/6(PQgoPQ) -> PQgoPQ/1
  PmiPQ/1 -> PQ Replay/2(PmiPQ)
  view/1(V) -> VF/1  "V"
  view/2(F) -> VF/2  "F"
  VtrefiPQ/1 -> PQ Replay/3(VtrefiPQ)
